simulink model "30_1_2018"  (R2024b)
settings: Solver=VariableStepAuto  StartTime=0.0  StopTime=10.0  RelTol=1e-3
settings Model: Creator=DT User  LastModifiedBy=DT User

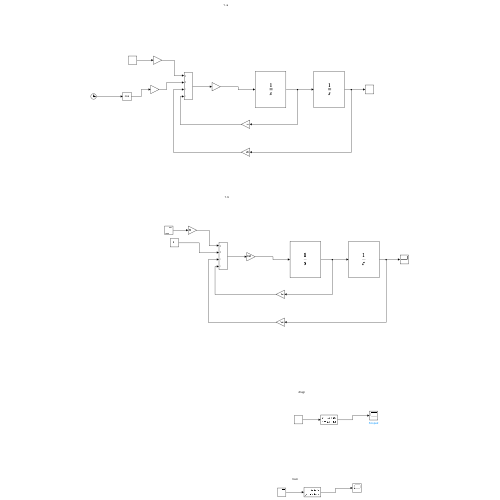
[thumbnail: Simulink's stored preview of the top-level diagram]
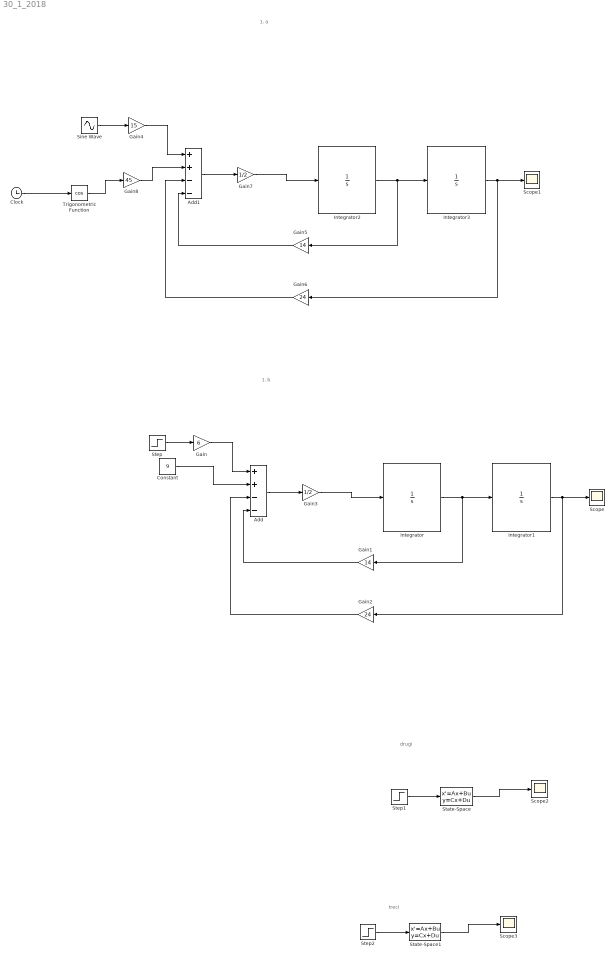
== system 30_1_2018 ==
  note: treci
  note: 1. a
  note: 1. b
  note: drugi
  Add : Sum  Inputs=++--
  Add1 : Sum  Inputs=++--
  Clock : Clock
  Constant : Constant  Value=9
  Gain : Gain  Gain=6
  Gain1 : Gain  Gain=14
  Gain2 : Gain  Gain=24
  Gain3 : Gain  Gain=1/2
  Gain4 : Gain  Gain=15
  Gain5 : Gain  Gain=14
  Gain6 : Gain  Gain=24
  Gain7 : Gain  Gain=1/2
  Gain8 : Gain  Gain=45
  Integrator : Integrator  InitialCondition=2
  Integrator1 : Integrator  InitialCondition=1
  Integrator2 : Integrator  InitialCondition=2
  Integrator3 : Integrator  InitialCondition=1
  Scope{,1..3} (4 alike) : Scope
  Sine Wave : Sin  SampleTime=0
  State-Space : StateSpace  A=[-1/10*0.01 0;0 0]  B=[10/10*0.01; 10/0.1]  C=[0 1]  D=0  InitialCondition=0
  State-Space1 : StateSpace  A=[0 1 0; 0 0 1; -1 -19 -8]  B=[0;0;5]  C=[5 0 0]  D=0  InitialCondition=0
  Step : Step  Time=0  SampleTime=0
  Step1 : Step  Time=0  SampleTime=0
  Step2 : Step  Time=0  SampleTime=0
  Trigonometric Function : Trigonometry  Operator=cos
  wires:
  Step/1 -> Gain/1
  Constant/1 -> Add/2
  Gain/1 -> Add/1
  Integrator/1 -> Gain1/1, Integrator1/1
  Gain3/1 -> Integrator/1
  Add/1 -> Gain3/1
  Gain1/1 -> Add/4
  Gain2/1 -> Add/3
  Integrator1/1 -> Scope/1, Gain2/1
  Integrator3/1 -> Gain6/1, Scope1/1
  Gain6/1 -> Add1/3
  Gain5/1 -> Add1/4
  Add1/1 -> Gain7/1
  Gain7/1 -> Integrator2/1
  Integrator2/1 -> Integrator3/1, Gain5/1
  Sine Wave/1 -> Gain4/1
  Gain4/1 -> Add1/1
  Clock/1 -> Trigonometric Function/1
  Trigonometric Function/1 -> Gain8/1
  Gain8/1 -> Add1/2
  State-Space/1 -> Scope2/1
  Step1/1 -> State-Space/1
  Step2/1 -> State-Space1/1
  State-Space1/1 -> Scope3/1
